simulink model "AsyncMachine"  (R2014a)
settings: Solver=ode23tb  StartTime=0.0  StopTime=10  RelTol=1e-3
libraries: powerlib x6
settings Model: Creator=ninad gaikawad  LastModifiedBy=ninad gaikawad
settings DebuggingCC: SolverPrmCheckMsg=none

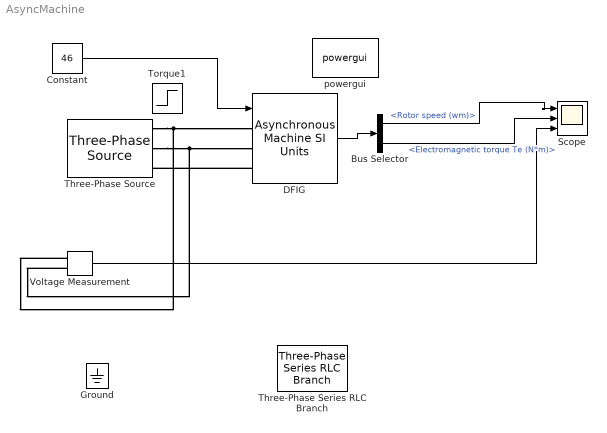
== system AsyncMachine ==
  Bus Selector : BusSelector  OutputSignals=Mechanical.Rotor speed (wm),Mechanical.Electromagnetic torque Te (N*m)
  Constant : Constant  Value=46
  DFIG : powerlib/Machines/Asynchronous Machine SI Units  PresetModel=No  MechanicalLoad=Torque Tm  ShowDetailedParameters=on  RotorType=Squirrel-cage  ReferenceFrame=Rotor  Units=SI  MeasurementBus=off  NominalParameters=[7.5e3 415 50]  Stator=[1.06 0.2065]  Rotor=[0.80 0.0810]  Cage1=[ 0.022 0.226/377]  Cage2=[ 0.022 0.226/377]  Lm=0.02135  Mechanical=[0.03 0.02187 3]  PolePairs=2  InitialConditions=[1 0 0 0 0 0 0 0]  SimulateSaturation=off  Saturation=[14.03593122, 27.81365428, 53.79336849, 72.68890987, 97.98006896, 148.6815601, 215.7428561, 302.9841135, 420.4778367 ; 230, 322, 414, 460, 506, 552, 598, 644, 690]  LoadFlowParameters=1492000  TsPowergui=0  TsBlock=-1  IterativeModel=Trapezoidal non iterative  Pmec=0
  Ground : powerlib/Elements/Ground  LConnTagsString=a
  Scope : Scope  NumInputPorts=3
      settings: YMin=-3225~0.0003075~-750  YMax=-3170~0.0003145~750
  Three-Phase Series RLC Branch : powerlib/Elements/Three-Phase Series RLC Branch  LConnTagsString=A|B|C  RConnTagsString=A|B|C  BranchType=R  Resistance=1  Inductance=1e-3  Capacitance=1e-6  Measurements=None
  Three-Phase Source : powerlib/Electrical Sources/Three-Phase Source  Voltage=415  PhaseAngle=0  Frequency=50  InternalConnection=Yg  SpecifyImpedance=off  Resistance=0  Inductance=0  ShortCircuitLevel=100e6  BaseVoltage=25e3  XRratio=7  BusType=swing  Pref=0  Qref=0  Qmin=-inf  Qmax=inf
  Torque1 : Step  Time=2  After=10  SampleTime=0
  Voltage Measurement : powerlib/Measurements/Voltage Measurement  PhasorSimulation=off  OutputType=Complex  PSBequivalent=0
  powergui : powerlib/powergui  Priority=1  SimulationMode=Continuous  SolverType=Tustin  SampleTime=50e-6  frequency=60  SPID=off  DisableSnubberDevices=off  DisableRonSwitches=off  DisableVfSwitches=off  SwTol=0  Interpol=off  DisplayEquations=off  Ts=0  methode=off  frequencyindice=50  Pbase=100e6  ErrMax=1e-4  Iterations=50  UnitsV=kV  UnitsW=MW  FunctionMessages=off  echomessages=off  HookPort=off  EnableUseOfTLC=off  x0status=blocks  RestoreLinks=warning  ResistiveCurrentMeasurement=off  Frange=[0:2:500]  Ylog=off  Xlog=on  ShowGrid=off  save=off  variable=ZData  structure=0  ZoomFFT=off  StartTime=0.0  cycles=1  DisplayStyle=1  fundamental=60  FreqAxis=off  MaxFrequency=1000  frequencyindicesteady=1  RmsSteady=1  display=off
  wires:
  Bus Selector/2 -> Scope/2  "<Electromagnetic torque Te (N*m)>"
  Voltage Measurement/1 -> Scope/3
  DFIG/1 -> Bus Selector/1
  Bus Selector/1 -> Scope/1  "<Rotor speed (wm)>"
  Constant/1 -> DFIG/1
  connections:
  Three-Phase Source/RConn1 -- Voltage Measurement/LConn1 -- DFIG/LConn1
  Three-Phase Source/RConn2 -- Voltage Measurement/LConn2 -- DFIG/LConn2
  DFIG/LConn3 -- Three-Phase Source/RConn3
